simulink model "DDCU_wxt_v03"  (R2014a)
settings: Solver=ode45  StartTime=0.0  StopTime=50  FixedStep=0.0005  RelTol=1e-3
values from neighbouring files (symbols this model uses):
  ag_thr = 0.4*g    (= 3.924)    [Veh_Par_wxt.m]
  B = 2.25    [Veh_Par_wxt.m]
  bra_pre_em = 12    [Veh_Par_wxt.m]
  bra_pre_gz2 = 12/3    (= 4)    [Veh_Par_wxt.m]
  bra_pre_gz34 = 12/3    (= 4)    [Veh_Par_wxt.m]
  bra_pre_yd = 12/2    (= 6)    [Veh_Par_wxt.m]
  brakepre_dem_data = [0 1 2 3 4 5 6 7 8 9 10 11 12]    [Veh_Par_wxt.m]
  brakeTrq_dem_data = [0 218.198 436.396 654.594 872.792 1090.99 1309.188 1527.386 1745.584 1963.782 2181.98 2400.178 2618.376]    [Veh_Par_wxt.m]
  bratrq_max = 4*2618.376    (= 10473.504)    [Veh_Par_wxt.m]
  eff_tran = 0.75    [Veh_Par_wxt.m]
  G = Mass*g    (= 36297)    [Veh_Par_wxt.m]
  kd1 = 1    [Veh_Par_wxt.m]
  kd2 = 1    [Veh_Par_wxt.m]
  kd3 = 1    [Veh_Par_wxt.m]
  ki1 = 1    [Veh_Par_wxt.m]
  ki2 = 1    [Veh_Par_wxt.m]
  ki3 = 1    [Veh_Par_wxt.m]
  kp1 = 1    [Veh_Par_wxt.m]
  kp2 = 1    [Veh_Par_wxt.m]
  kp3 = 1    [Veh_Par_wxt.m]
  L = 3.12    [Veh_Par_wxt.m]
  premax = 12    [Veh_Par_wxt.m]
  Radius = 0.20    (= 0.2)    [Veh_Par_wxt.m]
  s_opt_yi_add = 0.05    [Veh_Par_wxt.m]
  s_opt_zhuan_add = 0.05    [Veh_Par_wxt.m]
  spd_map_mot = [0 100 200 300 360 400 500 600 700 800 900]*tras_ratio    [Veh_Par_wxt.m]
  spdmax = 900*tras_ratio    (= 5580)    [Veh_Par_wxt.m]
  speed_thr_park = 5/3.6/Radius*30/pi    (= 66.3145596216)    [Veh_Par_wxt.m]
  tras_ratio = 6.2    [Veh_Par_wxt.m]
  trq_map_mot = [1200 1200 1200 1200 1200 1080 864 720 617 540 480]/tras_ratio    [Veh_Par_wxt.m]
  trqmax = 80    [Veh_Par_wxt.m]
  v_thr1_b = 5    [Veh_Par_wxt.m]
  v_thr2_b = 20    [Veh_Par_wxt.m]
  v_thr_park = 5    [Veh_Par_wxt.m]
undefined symbols (not defined in the file or in its folder): DiscIntNeverNeededParam
libraries: simulink x34, Solver_SF x1
(part 7 of 10)

== system DDCU_wxt_v03/MainControl/mode_control/backward/backward/Drive/驱动防滑控制TCS/直行TCS/直行/Subsystem1 ==
  brake_dem : Inport
  1-D Lookup Table : Lookup_n-D  NumberOfTableDimensions=1  BreakpointsForDimension1=brakeTrq_dem_data  Table=brakepre_dem_data  InternalRulePriority=Speed  RndMeth=Simplest  InputSameDT=on
  Constant : Constant  Value=bratrq_max
  Gain1 : Gain  Gain=1/2
  Gain2 : Gain  Gain=1/100
  Gain3 : Gain  Gain=1/2
  Product : Product
  brakepre_dem : Outport
  wires:
  brake_dem/1 -> Gain2/1
  Gain3/1 -> 1-D Lookup Table/1
  Gain2/1 -> Product/2
  Gain1/1 -> Gain3/1
  Product/1 -> Gain1/1
  Constant/1 -> Product/1
  1-D Lookup Table/1 -> brakepre_dem/1

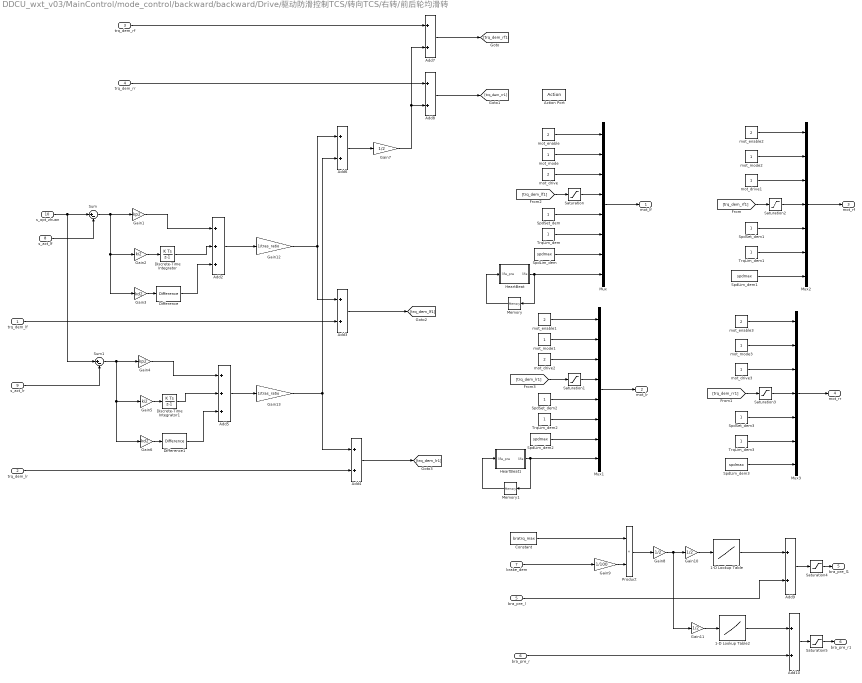
== system DDCU_wxt_v03/MainControl/mode_control/backward/backward/Drive/驱动防滑控制TCS/转向TCS/右转/前后轮均滑转 ==
  trq_dem_lf : Inport
  trq_dem_lr : Inport  Port=2
  trq_dem_rf : Inport  Port=3
  trq_dem_rr : Inport  Port=4
  bra_pre_l : Inport  Port=5
  bra_pre_r : Inport  Port=6
  brake_dem : Inport  Port=7
  s_act_lf : Inport  Port=8
  s_act_lr : Inport  Port=9
  s_opt_zhuan : Inport  Port=10
  Action Port : ActionPort
  1-D Lookup Table : Lookup_n-D  NumberOfTableDimensions=1  BreakpointsForDimension1=brakeTrq_dem_data  Table=brakepre_dem_data  InternalRulePriority=Speed  RndMeth=Simplest  InputSameDT=on
  1-D Lookup Table2 : Lookup_n-D  NumberOfTableDimensions=1  BreakpointsForDimension1=brakeTrq_dem_data  Table=brakepre_dem_data  InternalRulePriority=Speed  RndMeth=Simplest  InputSameDT=on
  Add{3..4,6..10} (7 alike) : Sum
  Add2 : Sum  Inputs=+++
  Add5 : Sum  Inputs=+++
  Constant : Constant  Value=bratrq_max
  Difference : simulink/Discrete/Difference  ICPrevInput=0.0  InputProcessing=Inherited  OutMin=[]  OutMax=[]  OutDataType=fixdt(1, 16)  OutScaling=2^-10  DoSatur=off
  Difference1 : simulink/Discrete/Difference  ICPrevInput=0.0  InputProcessing=Inherited  OutMin=[]  OutMax=[]  OutDataType=fixdt(1, 16)  OutScaling=2^-10  DoSatur=off
  Discrete-Time Integrator : DiscreteIntegrator  SampleTime=-1  ICPrevOutput=DiscIntNeverNeededParam  ICPrevScaledInput=DiscIntNeverNeededParam
  Discrete-Time Integrator1 : DiscreteIntegrator  SampleTime=-1  ICPrevOutput=DiscIntNeverNeededParam  ICPrevScaledInput=DiscIntNeverNeededParam
  Gain1 : Gain  Gain=kp2
  Gain{7..8,10..11} (4 alike) : Gain  Gain=1/2
  Gain12 : Gain  Gain=1/tras_ratio
  Gain13 : Gain  Gain=1/tras_ratio
  Gain2 : Gain  Gain=ki2
  Gain3 : Gain  Gain=kd2
  Gain4 : Gain  Gain=kp2
  Gain5 : Gain  Gain=ki2
  Gain6 : Gain  Gain=kd2
  Gain9 : Gain  Gain=1/100
  HeartBeat : MATLAB Function  TreatAsAtomicUnit=on
  HeartBeat1 : MATLAB Function  TreatAsAtomicUnit=on
  Memory : Memory  InheritSampleTime=on
  Memory1 : Memory  InheritSampleTime=on
  Mux : Mux  Inputs=8
  Mux1 : Mux  Inputs=8
  Mux2 : Mux  Inputs=7
  Mux3 : Mux  Inputs=7
  Product : Product
  Saturation{,1..3} (4 alike) : Saturate  UpperLimit=trqmax  LowerLimit=-trqmax
  Saturation4 : Saturate  UpperLimit=premax  LowerLimit=0
  Saturation5 : Saturate  UpperLimit=premax  LowerLimit=0
  SpdLim_dem{,1..3} (4 alike) : Constant  Value=spdmax
  SpdSet_dem{,1..3} (4 alike) : Constant
  Sum : Sum  Inputs=|+-
  Sum1 : Sum  Inputs=|+-
  TrqLim_dem{,1..3} (4 alike) : Constant
  mot_drive : Constant  Value=2
  mot_drive1 : Constant
  mot_drive2 : Constant  Value=2
  mot_drive3 : Constant
  mot_enable{,1..3} (4 alike) : Constant  Value=2
  mot_mode{,1..3} (4 alike) : Constant
  mot_lf : Outport
  mot_lr : Outport  Port=2
  mot_rf : Outport  Port=3
  mot_rr : Outport  Port=4
  bra_pre_l1 : Outport  Port=5
  bra_pre_r1 : Outport  Port=6
  wires:
  Saturation5/1 -> bra_pre_r1/1
  Saturation4/1 -> bra_pre_l1/1
  Saturation3/1 -> Mux3/4
  Saturation2/1 -> Mux2/4
  Saturation1/1 -> Mux1/4
  Saturation/1 -> Mux/4
  Difference1/1 -> Add5/3
  Discrete-Time Integrator1/1 -> Add5/2
  Difference/1 -> Add2/3
  Discrete-Time Integrator/1 -> Add2/2
  Gain3/1 -> Difference/1
  brake_dem/1 -> Gain9/1
  Add10/1 -> Saturation5/1
  bra_pre_r/1 -> Add10/2
  1-D Lookup Table2/1 -> Add10/1
  Gain11/1 -> 1-D Lookup Table2/1
  Gain10/1 -> 1-D Lookup Table/1
  Gain9/1 -> Product/2
  Gain8/1 -> Gain10/1, Gain11/1
  Product/1 -> Gain8/1
  Constant/1 -> Product/1
  1-D Lookup Table/1 -> Add9/1
  Add9/1 -> Saturation4/1
  bra_pre_l/1 -> Add9/2
  SpdLim_dem3/1 -> Mux3/7
  TrqLim_dem3/1 -> Mux3/6
  Mux3/1 -> mot_rr/1
  SpdSet_dem3/1 -> Mux3/5
  mot_enable3/1 -> Mux3/1
  [trq_dem_rr1] -> Saturation3/1
  mot_mode3/1 -> Mux3/2
  mot_drive3/1 -> Mux3/3
  SpdLim_dem2/1 -> Mux1/7
  Memory1/1 -> HeartBeat1/1(life_pre)
  HeartBeat1/1(life) -> Memory1/1, Mux1/8
  TrqLim_dem2/1 -> Mux1/6
  Mux1/1 -> mot_lr/1
  SpdSet_dem2/1 -> Mux1/5
  mot_enable1/1 -> Mux1/1
  [trq_dem_lr1] -> Saturation1/1
  mot_mode1/1 -> Mux1/2
  mot_drive2/1 -> Mux1/3
  SpdLim_dem1/1 -> Mux2/7
  TrqLim_dem1/1 -> Mux2/6
  Mux2/1 -> mot_rf/1
  SpdSet_dem1/1 -> Mux2/5
  mot_enable2/1 -> Mux2/1
  [trq_dem_rf1] -> Saturation2/1
  mot_mode2/1 -> Mux2/2
  mot_drive1/1 -> Mux2/3
  SpdLim_dem/1 -> Mux/7
  Memory/1 -> HeartBeat/1(life_pre)
  HeartBeat/1(life) -> Memory/1, Mux/8
  TrqLim_dem/1 -> Mux/6
  Mux/1 -> mot_lf/1
  SpdSet_dem/1 -> Mux/5
  mot_enable/1 -> Mux/1
  [trq_dem_lf1] -> Saturation/1
  mot_mode/1 -> Mux/2
  mot_drive/1 -> Mux/3
  s_opt_zhuan/1 -> Sum1/1, Sum/1
  Sum/1 -> Gain2/1, Gain3/1, Gain1/1
  Gain1/1 -> Add2/1
  Gain2/1 -> Discrete-Time Integrator/1
  s_act_lf/1 -> Sum/2
  Add2/1 -> Gain12/1
  trq_dem_lf/1 -> Add3/2
  Add3/1 -> [trq_dem_lf1]
  Add4/1 -> [trq_dem_lr1]
  Sum1/1 -> Gain5/1, Gain6/1, Gain4/1
  Gain4/1 -> Add5/1
  Gain5/1 -> Discrete-Time Integrator1/1
  Gain6/1 -> Difference1/1
  s_act_lr/1 -> Sum1/2
  Add5/1 -> Gain13/1
  trq_dem_lr/1 -> Add4/2
  Add6/1 -> Gain7/1
  trq_dem_rf/1 -> Add7/1
  Gain7/1 -> Add8/2, Add7/2
  Add7/1 -> [trq_dem_rf1]
  trq_dem_rr/1 -> Add8/1
  Add8/1 -> [trq_dem_rr1]
  Gain12/1 -> Add3/1, Add6/1
  Gain13/1 -> Add4/1, Add6/2

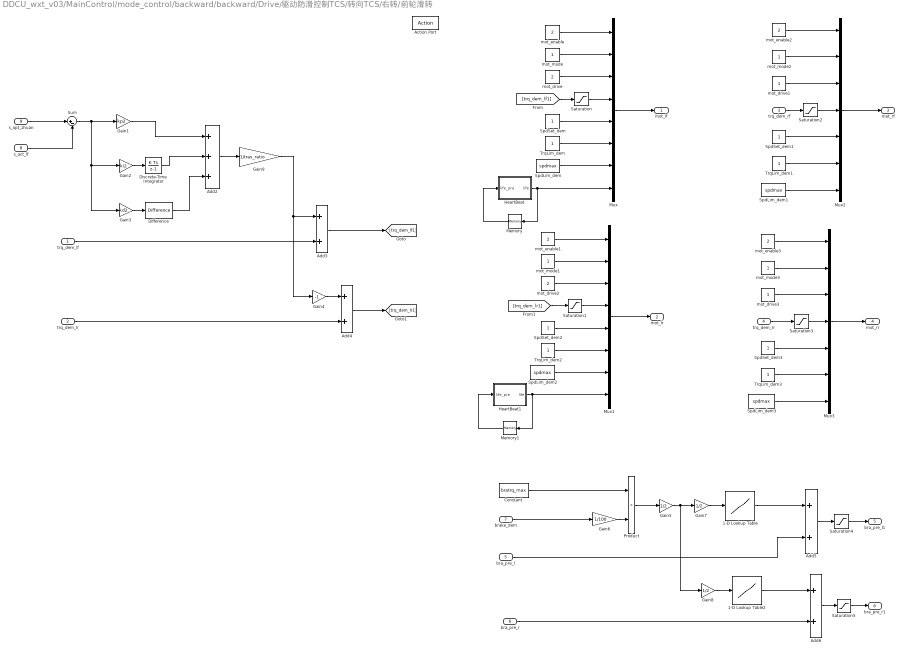
== system DDCU_wxt_v03/MainControl/mode_control/backward/backward/Drive/驱动防滑控制TCS/转向TCS/右转/前轮滑转 ==
  trq_dem_lf : Inport
  trq_dem_lr : Inport  Port=2
  trq_dem_rf : Inport  Port=3
  trq_dem_rr : Inport  Port=4
  bra_pre_l : Inport  Port=5
  bra_pre_r : Inport  Port=6
  brake_dem : Inport  Port=7
  s_act_lf : Inport  Port=8
  s_opt_zhuan : Inport  Port=9
  Action Port : ActionPort
  1-D Lookup Table : Lookup_n-D  NumberOfTableDimensions=1  BreakpointsForDimension1=brakeTrq_dem_data  Table=brakepre_dem_data  InternalRulePriority=Speed  RndMeth=Simplest  InputSameDT=on
  1-D Lookup Table2 : Lookup_n-D  NumberOfTableDimensions=1  BreakpointsForDimension1=brakeTrq_dem_data  Table=brakepre_dem_data  InternalRulePriority=Speed  RndMeth=Simplest  InputSameDT=on
  Add2 : Sum  Inputs=+++
  Add{3..6} (4 alike) : Sum
  Constant : Constant  Value=bratrq_max
  Difference : simulink/Discrete/Difference  ICPrevInput=0.0  InputProcessing=Inherited  OutMin=[]  OutMax=[]  OutDataType=fixdt(1, 16)  OutScaling=2^-10  DoSatur=off
  Discrete-Time Integrator : DiscreteIntegrator  SampleTime=-1  ICPrevOutput=DiscIntNeverNeededParam  ICPrevScaledInput=DiscIntNeverNeededParam
  Gain1 : Gain  Gain=kp2
  Gain2 : Gain  Gain=ki2
  Gain3 : Gain  Gain=kd2
  Gain4 : Gain  Gain=-1
  Gain5 : Gain  Gain=1/2
  Gain6 : Gain  Gain=1/100
  Gain7 : Gain  Gain=1/2
  Gain8 : Gain  Gain=1/2
  Gain9 : Gain  Gain=1/tras_ratio
  HeartBeat : MATLAB Function  TreatAsAtomicUnit=on
  HeartBeat1 : MATLAB Function  TreatAsAtomicUnit=on
  Memory : Memory  InheritSampleTime=on
  Memory1 : Memory  InheritSampleTime=on
  Mux : Mux  Inputs=8
  Mux1 : Mux  Inputs=8
  Mux2 : Mux  Inputs=7
  Mux3 : Mux  Inputs=7
  Product : Product
  Saturation{,1..3} (4 alike) : Saturate  UpperLimit=trqmax  LowerLimit=-trqmax
  Saturation4 : Saturate  UpperLimit=premax  LowerLimit=0
  Saturation5 : Saturate  UpperLimit=premax  LowerLimit=0
  SpdLim_dem{,1..3} (4 alike) : Constant  Value=spdmax
  SpdSet_dem{,1..3} (4 alike) : Constant
  Sum : Sum  Inputs=|+-
  TrqLim_dem{,1..3} (4 alike) : Constant
  mot_drive : Constant  Value=2
  mot_drive1 : Constant
  mot_drive2 : Constant  Value=2
  mot_drive3 : Constant
  mot_enable{,1..3} (4 alike) : Constant  Value=2
  mot_mode{,1..3} (4 alike) : Constant
  mot_lf : Outport
  mot_lr : Outport  Port=2
  mot_rf : Outport  Port=3
  mot_rr : Outport  Port=4
  bra_pre_l1 : Outport  Port=5
  bra_pre_r1 : Outport  Port=6
  wires:
  Saturation5/1 -> bra_pre_r1/1
  Saturation4/1 -> bra_pre_l1/1
  Saturation3/1 -> Mux3/4
  Saturation2/1 -> Mux2/4
  Saturation1/1 -> Mux1/4
  Saturation/1 -> Mux/4
  Difference/1 -> Add2/3
  Discrete-Time Integrator/1 -> Add2/2
  brake_dem/1 -> Gain6/1
  Add6/1 -> Saturation5/1
  bra_pre_r/1 -> Add6/2
  1-D Lookup Table2/1 -> Add6/1
  Gain8/1 -> 1-D Lookup Table2/1
  Gain7/1 -> 1-D Lookup Table/1
  Gain6/1 -> Product/2
  Gain5/1 -> Gain7/1, Gain8/1
  Product/1 -> Gain5/1
  Constant/1 -> Product/1
  1-D Lookup Table/1 -> Add5/1
  Add5/1 -> Saturation4/1
  bra_pre_l/1 -> Add5/2
  SpdLim_dem3/1 -> Mux3/7
  TrqLim_dem3/1 -> Mux3/6
  Mux3/1 -> mot_rr/1
  SpdSet_dem3/1 -> Mux3/5
  mot_enable3/1 -> Mux3/1
  trq_dem_rr/1 -> Saturation3/1
  mot_mode3/1 -> Mux3/2
  mot_drive3/1 -> Mux3/3
  SpdLim_dem2/1 -> Mux1/7
  Memory1/1 -> HeartBeat1/1(life_pre)
  HeartBeat1/1(life) -> Memory1/1, Mux1/8
  TrqLim_dem2/1 -> Mux1/6
  Mux1/1 -> mot_lr/1
  SpdSet_dem2/1 -> Mux1/5
  mot_enable1/1 -> Mux1/1
  [trq_dem_lr1] -> Saturation1/1
  mot_mode1/1 -> Mux1/2
  mot_drive2/1 -> Mux1/3
  SpdLim_dem1/1 -> Mux2/7
  TrqLim_dem1/1 -> Mux2/6
  Mux2/1 -> mot_rf/1
  SpdSet_dem1/1 -> Mux2/5
  mot_enable2/1 -> Mux2/1
  trq_dem_rf/1 -> Saturation2/1
  mot_mode2/1 -> Mux2/2
  mot_drive1/1 -> Mux2/3
  SpdLim_dem/1 -> Mux/7
  Memory/1 -> HeartBeat/1(life_pre)
  HeartBeat/1(life) -> Memory/1, Mux/8
  TrqLim_dem/1 -> Mux/6
  Mux/1 -> mot_lf/1
  SpdSet_dem/1 -> Mux/5
  mot_enable/1 -> Mux/1
  [trq_dem_lf1] -> Saturation/1
  mot_mode/1 -> Mux/2
  mot_drive/1 -> Mux/3
  s_opt_zhuan/1 -> Sum/1
  Sum/1 -> Gain2/1, Gain3/1, Gain1/1
  Gain1/1 -> Add2/1
  Gain2/1 -> Discrete-Time Integrator/1
  Gain3/1 -> Difference/1
  s_act_lf/1 -> Sum/2
  Add2/1 -> Gain9/1
  trq_dem_lf/1 -> Add3/2
  Add3/1 -> [trq_dem_lf1]
  Gain4/1 -> Add4/1
  trq_dem_lr/1 -> Add4/2
  Add4/1 -> [trq_dem_lr1]
  Gain9/1 -> Gain4/1, Add3/1

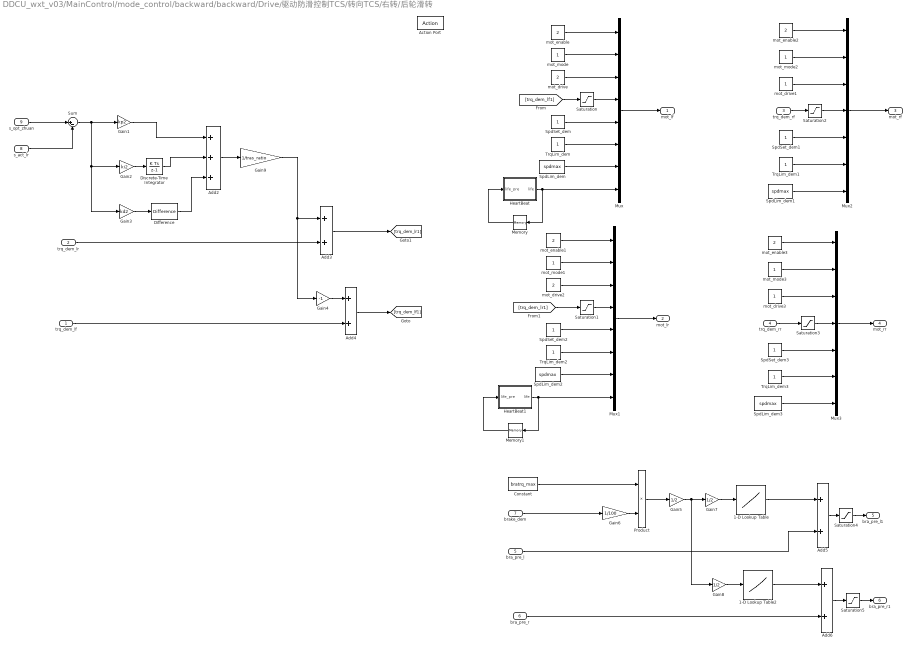
== system DDCU_wxt_v03/MainControl/mode_control/backward/backward/Drive/驱动防滑控制TCS/转向TCS/右转/后轮滑转 ==
  trq_dem_lf : Inport
  trq_dem_lr : Inport  Port=2
  trq_dem_rf : Inport  Port=3
  trq_dem_rr : Inport  Port=4
  bra_pre_l : Inport  Port=5
  bra_pre_r : Inport  Port=6
  brake_dem : Inport  Port=7
  s_act_lr : Inport  Port=8
  s_opt_zhuan : Inport  Port=9
  Action Port : ActionPort
  1-D Lookup Table : Lookup_n-D  NumberOfTableDimensions=1  BreakpointsForDimension1=brakeTrq_dem_data  Table=brakepre_dem_data  InternalRulePriority=Speed  RndMeth=Simplest  InputSameDT=on
  1-D Lookup Table2 : Lookup_n-D  NumberOfTableDimensions=1  BreakpointsForDimension1=brakeTrq_dem_data  Table=brakepre_dem_data  InternalRulePriority=Speed  RndMeth=Simplest  InputSameDT=on
  Add2 : Sum  Inputs=+++
  Add{3..6} (4 alike) : Sum
  Constant : Constant  Value=bratrq_max
  Difference : simulink/Discrete/Difference  ICPrevInput=0.0  InputProcessing=Inherited  OutMin=[]  OutMax=[]  OutDataType=fixdt(1, 16)  OutScaling=2^-10  DoSatur=off
  Discrete-Time Integrator : DiscreteIntegrator  SampleTime=-1  ICPrevOutput=DiscIntNeverNeededParam  ICPrevScaledInput=DiscIntNeverNeededParam
  Gain1 : Gain  Gain=kp2
  Gain2 : Gain  Gain=ki2
  Gain3 : Gain  Gain=kd2
  Gain4 : Gain  Gain=-1
  Gain5 : Gain  Gain=1/2
  Gain6 : Gain  Gain=1/100
  Gain7 : Gain  Gain=1/2
  Gain8 : Gain  Gain=1/2
  Gain9 : Gain  Gain=1/tras_ratio
  HeartBeat : MATLAB Function  TreatAsAtomicUnit=on
  HeartBeat1 : MATLAB Function  TreatAsAtomicUnit=on
  Memory : Memory  InheritSampleTime=on
  Memory1 : Memory  InheritSampleTime=on
  Mux : Mux  Inputs=8
  Mux1 : Mux  Inputs=8
  Mux2 : Mux  Inputs=7
  Mux3 : Mux  Inputs=7
  Product : Product
  Saturation{,1..3} (4 alike) : Saturate  UpperLimit=trqmax  LowerLimit=-trqmax
  Saturation4 : Saturate  UpperLimit=premax  LowerLimit=0
  Saturation5 : Saturate  UpperLimit=premax  LowerLimit=0
  SpdLim_dem{,1..3} (4 alike) : Constant  Value=spdmax
  SpdSet_dem{,1..3} (4 alike) : Constant
  Sum : Sum  Inputs=|+-
  TrqLim_dem{,1..3} (4 alike) : Constant
  mot_drive : Constant  Value=2
  mot_drive1 : Constant
  mot_drive2 : Constant  Value=2
  mot_drive3 : Constant
  mot_enable{,1..3} (4 alike) : Constant  Value=2
  mot_mode{,1..3} (4 alike) : Constant
  mot_lf : Outport
  mot_lr : Outport  Port=2
  mot_rf : Outport  Port=3
  mot_rr : Outport  Port=4
  bra_pre_l1 : Outport  Port=5
  bra_pre_r1 : Outport  Port=6
  wires:
  Saturation5/1 -> bra_pre_r1/1
  Saturation4/1 -> bra_pre_l1/1
  Saturation3/1 -> Mux3/4
  Saturation2/1 -> Mux2/4
  Saturation1/1 -> Mux1/4
  Saturation/1 -> Mux/4
  Difference/1 -> Add2/3
  Discrete-Time Integrator/1 -> Add2/2
  brake_dem/1 -> Gain6/1
  Add6/1 -> Saturation5/1
  bra_pre_r/1 -> Add6/2
  1-D Lookup Table2/1 -> Add6/1
  Gain8/1 -> 1-D Lookup Table2/1
  Gain7/1 -> 1-D Lookup Table/1
  Gain6/1 -> Product/2
  Gain5/1 -> Gain7/1, Gain8/1
  Product/1 -> Gain5/1
  Constant/1 -> Product/1
  1-D Lookup Table/1 -> Add5/1
  Add5/1 -> Saturation4/1
  bra_pre_l/1 -> Add5/2
  Add4/1 -> [trq_dem_lf1]
  trq_dem_lf/1 -> Add4/2
  Gain4/1 -> Add4/1
  Add3/1 -> [trq_dem_lr1]
  trq_dem_lr/1 -> Add3/2
  Add2/1 -> Gain9/1
  s_act_lr/1 -> Sum/2
  Gain3/1 -> Difference/1
  Gain2/1 -> Discrete-Time Integrator/1
  Gain1/1 -> Add2/1
  Sum/1 -> Gain1/1, Gain3/1, Gain2/1
  s_opt_zhuan/1 -> Sum/1
  mot_drive/1 -> Mux/3
  mot_mode/1 -> Mux/2
  [trq_dem_lf1] -> Saturation/1
  mot_enable/1 -> Mux/1
  SpdSet_dem/1 -> Mux/5
  Mux/1 -> mot_lf/1
  TrqLim_dem/1 -> Mux/6
  HeartBeat/1(life) -> Mux/8, Memory/1
  Memory/1 -> HeartBeat/1(life_pre)
  SpdLim_dem/1 -> Mux/7
  mot_drive1/1 -> Mux2/3
  mot_mode2/1 -> Mux2/2
  trq_dem_rf/1 -> Saturation2/1
  mot_enable2/1 -> Mux2/1
  SpdSet_dem1/1 -> Mux2/5
  Mux2/1 -> mot_rf/1
  TrqLim_dem1/1 -> Mux2/6
  SpdLim_dem1/1 -> Mux2/7
  mot_drive2/1 -> Mux1/3
  mot_mode1/1 -> Mux1/2
  [trq_dem_lr1] -> Saturation1/1
  mot_enable1/1 -> Mux1/1
  SpdSet_dem2/1 -> Mux1/5
  Mux1/1 -> mot_lr/1
  TrqLim_dem2/1 -> Mux1/6
  HeartBeat1/1(life) -> Mux1/8, Memory1/1
  Memory1/1 -> HeartBeat1/1(life_pre)
  SpdLim_dem2/1 -> Mux1/7
  mot_drive3/1 -> Mux3/3
  mot_mode3/1 -> Mux3/2
  trq_dem_rr/1 -> Saturation3/1
  mot_enable3/1 -> Mux3/1
  SpdSet_dem3/1 -> Mux3/5
  Mux3/1 -> mot_rr/1
  TrqLim_dem3/1 -> Mux3/6
  SpdLim_dem3/1 -> Mux3/7
  Gain9/1 -> Add3/1, Gain4/1

== system DDCU_wxt_v03/MainControl/mode_control/backward/backward/Drive/驱动防滑控制TCS/转向TCS/右转/无滑转 ==
  trq_dem_lf : Inport
  trq_dem_lr : Inport  Port=2
  trq_dem_rf : Inport  Port=3
  trq_dem_rr : Inport  Port=4
  bra_pre_l : Inport  Port=5
  bra_pre_r : Inport  Port=6
  brake_dem : Inport  Port=7
  Action Port : ActionPort
  1-D Lookup Table : Lookup_n-D  NumberOfTableDimensions=1  BreakpointsForDimension1=brakeTrq_dem_data  Table=brakepre_dem_data  InternalRulePriority=Speed  RndMeth=Simplest  InputSameDT=on
  1-D Lookup Table2 : Lookup_n-D  NumberOfTableDimensions=1  BreakpointsForDimension1=brakeTrq_dem_data  Table=brakepre_dem_data  InternalRulePriority=Speed  RndMeth=Simplest  InputSameDT=on
  Add2 : Sum
  Add3 : Sum
  Constant : Constant  Value=bratrq_max
  Gain1 : Gain  Gain=1/2
  Gain2 : Gain  Gain=1/100
  Gain3 : Gain  Gain=1/2
  Gain4 : Gain  Gain=1/2
  HeartBeat : MATLAB Function  TreatAsAtomicUnit=on
  HeartBeat1 : MATLAB Function  TreatAsAtomicUnit=on
  Memory : Memory  InheritSampleTime=on
  Memory1 : Memory  InheritSampleTime=on
  Mux : Mux  Inputs=8
  Mux1 : Mux  Inputs=8
  Mux2 : Mux  Inputs=7
  Mux3 : Mux  Inputs=7
  Product : Product
  Saturation{,1..3} (4 alike) : Saturate  UpperLimit=trqmax  LowerLimit=-trqmax
  Saturation4 : Saturate  UpperLimit=premax  LowerLimit=0
  Saturation5 : Saturate  UpperLimit=premax  LowerLimit=0
  SpdLim_dem{,1..3} (4 alike) : Constant  Value=spdmax
  SpdSet_dem{,1..3} (4 alike) : Constant
  TrqLim_dem{,1..3} (4 alike) : Constant
  mot_drive : Constant  Value=2
  mot_drive1 : Constant
  mot_drive2 : Constant  Value=2
  mot_drive3 : Constant
  mot_enable{,1..3} (4 alike) : Constant  Value=2
  mot_mode{,1..3} (4 alike) : Constant
  mot_lf : Outport
  mot_lr : Outport  Port=2
  mot_rf : Outport  Port=3
  mot_rr : Outport  Port=4
  bra_pre_l1 : Outport  Port=5
  bra_pre_r1 : Outport  Port=6
  wires:
  Saturation5/1 -> bra_pre_r1/1
  Saturation4/1 -> bra_pre_l1/1
  Saturation3/1 -> Mux3/4
  Saturation2/1 -> Mux2/4
  Saturation1/1 -> Mux1/4
  Saturation/1 -> Mux/4
  brake_dem/1 -> Gain2/1
  Add3/1 -> Saturation5/1
  bra_pre_r/1 -> Add3/2
  1-D Lookup Table2/1 -> Add3/1
  Gain4/1 -> 1-D Lookup Table2/1
  Gain3/1 -> 1-D Lookup Table/1
  Gain2/1 -> Product/2
  Gain1/1 -> Gain3/1, Gain4/1
  Product/1 -> Gain1/1
  Constant/1 -> Product/1
  1-D Lookup Table/1 -> Add2/1
  Add2/1 -> Saturation4/1
  bra_pre_l/1 -> Add2/2
  mot_drive/1 -> Mux/3
  mot_mode/1 -> Mux/2
  trq_dem_lf/1 -> Saturation/1
  mot_enable/1 -> Mux/1
  SpdSet_dem/1 -> Mux/5
  Mux/1 -> mot_lf/1
  TrqLim_dem/1 -> Mux/6
  HeartBeat/1(life) -> Mux/8, Memory/1
  Memory/1 -> HeartBeat/1(life_pre)
  SpdLim_dem/1 -> Mux/7
  mot_drive1/1 -> Mux2/3
  mot_mode2/1 -> Mux2/2
  trq_dem_rf/1 -> Saturation2/1
  mot_enable2/1 -> Mux2/1
  SpdSet_dem1/1 -> Mux2/5
  Mux2/1 -> mot_rf/1
  TrqLim_dem1/1 -> Mux2/6
  SpdLim_dem1/1 -> Mux2/7
  mot_drive2/1 -> Mux1/3
  mot_mode1/1 -> Mux1/2
  trq_dem_lr/1 -> Saturation1/1
  mot_enable1/1 -> Mux1/1
  SpdSet_dem2/1 -> Mux1/5
  Mux1/1 -> mot_lr/1
  TrqLim_dem2/1 -> Mux1/6
  HeartBeat1/1(life) -> Mux1/8, Memory1/1
  Memory1/1 -> HeartBeat1/1(life_pre)
  SpdLim_dem2/1 -> Mux1/7
  mot_drive3/1 -> Mux3/3
  mot_mode3/1 -> Mux3/2
  trq_dem_rr/1 -> Saturation3/1
  mot_enable3/1 -> Mux3/1
  SpdSet_dem3/1 -> Mux3/5
  Mux3/1 -> mot_rr/1
  TrqLim_dem3/1 -> Mux3/6
  SpdLim_dem3/1 -> Mux3/7

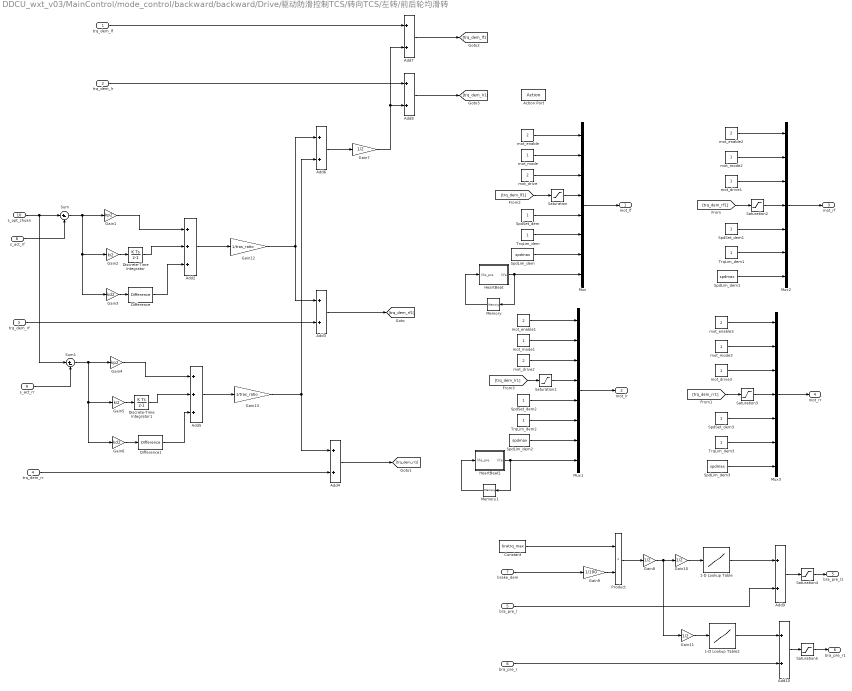
== system DDCU_wxt_v03/MainControl/mode_control/backward/backward/Drive/驱动防滑控制TCS/转向TCS/左转/前后轮均滑转 ==
  trq_dem_lf : Inport
  trq_dem_lr : Inport  Port=2
  trq_dem_rf : Inport  Port=3
  trq_dem_rr : Inport  Port=4
  bra_pre_l : Inport  Port=5
  bra_pre_r : Inport  Port=6
  brake_dem : Inport  Port=7
  s_act_rf : Inport  Port=8
  s_act_rr : Inport  Port=9
  s_opt_zhuan : Inport  Port=10
  Action Port : ActionPort
  1-D Lookup Table : Lookup_n-D  NumberOfTableDimensions=1  BreakpointsForDimension1=brakeTrq_dem_data  Table=brakepre_dem_data  InternalRulePriority=Speed  RndMeth=Simplest  InputSameDT=on
  1-D Lookup Table2 : Lookup_n-D  NumberOfTableDimensions=1  BreakpointsForDimension1=brakeTrq_dem_data  Table=brakepre_dem_data  InternalRulePriority=Speed  RndMeth=Simplest  InputSameDT=on
  Add{3..4,6..10} (7 alike) : Sum
  Add2 : Sum  Inputs=+++
  Add5 : Sum  Inputs=+++
  Constant : Constant  Value=bratrq_max
  Difference : simulink/Discrete/Difference  ICPrevInput=0.0  InputProcessing=Inherited  OutMin=[]  OutMax=[]  OutDataType=fixdt(1, 16)  OutScaling=2^-10  DoSatur=off
  Difference1 : simulink/Discrete/Difference  ICPrevInput=0.0  InputProcessing=Inherited  OutMin=[]  OutMax=[]  OutDataType=fixdt(1, 16)  OutScaling=2^-10  DoSatur=off
  Discrete-Time Integrator : DiscreteIntegrator  SampleTime=-1  ICPrevOutput=DiscIntNeverNeededParam  ICPrevScaledInput=DiscIntNeverNeededParam
  Discrete-Time Integrator1 : DiscreteIntegrator  SampleTime=-1  ICPrevOutput=DiscIntNeverNeededParam  ICPrevScaledInput=DiscIntNeverNeededParam
  Gain1 : Gain  Gain=kp2
  Gain{7..8,10..11} (4 alike) : Gain  Gain=1/2
  Gain12 : Gain  Gain=1/tras_ratio
  Gain13 : Gain  Gain=1/tras_ratio
  Gain2 : Gain  Gain=ki2
  Gain3 : Gain  Gain=kd2
  Gain4 : Gain  Gain=kp2
  Gain5 : Gain  Gain=ki2
  Gain6 : Gain  Gain=kd2
  Gain9 : Gain  Gain=1/100
  HeartBeat : MATLAB Function  TreatAsAtomicUnit=on
  HeartBeat1 : MATLAB Function  TreatAsAtomicUnit=on
  Memory : Memory  InheritSampleTime=on
  Memory1 : Memory  InheritSampleTime=on
  Mux : Mux  Inputs=8
  Mux1 : Mux  Inputs=8
  Mux2 : Mux  Inputs=7
  Mux3 : Mux  Inputs=7
  Product : Product
  Saturation{,1..3} (4 alike) : Saturate  UpperLimit=trqmax  LowerLimit=-trqmax
  Saturation4 : Saturate  UpperLimit=premax  LowerLimit=0
  Saturation5 : Saturate  UpperLimit=premax  LowerLimit=0
  SpdLim_dem{,1..3} (4 alike) : Constant  Value=spdmax
  SpdSet_dem{,1..3} (4 alike) : Constant
  Sum : Sum  Inputs=|+-
  Sum1 : Sum  Inputs=|+-
  TrqLim_dem{,1..3} (4 alike) : Constant
  mot_drive : Constant  Value=2
  mot_drive1 : Constant
  mot_drive2 : Constant  Value=2
  mot_drive3 : Constant
  mot_enable{,1..3} (4 alike) : Constant  Value=2
  mot_mode{,1..3} (4 alike) : Constant
  mot_lf : Outport
  mot_lr : Outport  Port=2
  mot_rf : Outport  Port=3
  mot_rr : Outport  Port=4
  bra_pre_l1 : Outport  Port=5
  bra_pre_r1 : Outport  Port=6
  wires:
  Saturation5/1 -> bra_pre_r1/1
  Saturation4/1 -> bra_pre_l1/1
  Saturation3/1 -> Mux3/4
  Saturation2/1 -> Mux2/4
  Saturation1/1 -> Mux1/4
  Saturation/1 -> Mux/4
  Difference1/1 -> Add5/3
  Discrete-Time Integrator1/1 -> Add5/2
  Difference/1 -> Add2/3
  Discrete-Time Integrator/1 -> Add2/2
  brake_dem/1 -> Gain9/1
  Add10/1 -> Saturation5/1
  bra_pre_r/1 -> Add10/2
  1-D Lookup Table2/1 -> Add10/1
  Gain11/1 -> 1-D Lookup Table2/1
  Gain10/1 -> 1-D Lookup Table/1
  Gain9/1 -> Product/2
  Gain8/1 -> Gain10/1, Gain11/1
  Product/1 -> Gain8/1
  Constant/1 -> Product/1
  1-D Lookup Table/1 -> Add9/1
  Add9/1 -> Saturation4/1
  bra_pre_l/1 -> Add9/2
  Add8/1 -> [trq_dem_lr1]
  trq_dem_lr/1 -> Add8/1
  Add7/1 -> [trq_dem_lf1]
  Gain7/1 -> Add7/2, Add8/2
  trq_dem_lf/1 -> Add7/1
  Add6/1 -> Gain7/1
  trq_dem_rr/1 -> Add4/2
  Add5/1 -> Gain13/1
  s_act_rr/1 -> Sum1/2
  Gain6/1 -> Difference1/1
  Gain5/1 -> Discrete-Time Integrator1/1
  Gain4/1 -> Add5/1
  Sum1/1 -> Gain4/1, Gain6/1, Gain5/1
  Add4/1 -> [trq_dem_rr1]
  Add3/1 -> [trq_dem_rf1]
  trq_dem_rf/1 -> Add3/2
  Add2/1 -> Gain12/1
  s_act_rf/1 -> Sum/2
  Gain3/1 -> Difference/1
  Gain2/1 -> Discrete-Time Integrator/1
  Gain1/1 -> Add2/1
  Sum/1 -> Gain1/1, Gain3/1, Gain2/1
  s_opt_zhuan/1 -> Sum/1, Sum1/1
  mot_drive/1 -> Mux/3
  mot_mode/1 -> Mux/2
  [trq_dem_lf1] -> Saturation/1
  mot_enable/1 -> Mux/1
  SpdSet_dem/1 -> Mux/5
  Mux/1 -> mot_lf/1
  TrqLim_dem/1 -> Mux/6
  HeartBeat/1(life) -> Mux/8, Memory/1
  Memory/1 -> HeartBeat/1(life_pre)
  SpdLim_dem/1 -> Mux/7
  mot_drive1/1 -> Mux2/3
  mot_mode2/1 -> Mux2/2
  [trq_dem_rf1] -> Saturation2/1
  mot_enable2/1 -> Mux2/1
  SpdSet_dem1/1 -> Mux2/5
  Mux2/1 -> mot_rf/1
  TrqLim_dem1/1 -> Mux2/6
  SpdLim_dem1/1 -> Mux2/7
  mot_drive2/1 -> Mux1/3
  mot_mode1/1 -> Mux1/2
  [trq_dem_lr1] -> Saturation1/1
  mot_enable1/1 -> Mux1/1
  SpdSet_dem2/1 -> Mux1/5
  Mux1/1 -> mot_lr/1
  TrqLim_dem2/1 -> Mux1/6
  HeartBeat1/1(life) -> Mux1/8, Memory1/1
  Memory1/1 -> HeartBeat1/1(life_pre)
  SpdLim_dem2/1 -> Mux1/7
  mot_drive3/1 -> Mux3/3
  mot_mode3/1 -> Mux3/2
  [trq_dem_rr1] -> Saturation3/1
  mot_enable3/1 -> Mux3/1
  SpdSet_dem3/1 -> Mux3/5
  Mux3/1 -> mot_rr/1
  TrqLim_dem3/1 -> Mux3/6
  SpdLim_dem3/1 -> Mux3/7
  Gain12/1 -> Add6/1, Add3/1
  Gain13/1 -> Add6/2, Add4/1

== system DDCU_wxt_v03/MainControl/mode_control/backward/backward/Drive/驱动防滑控制TCS/转向TCS/左转/前轮滑转 ==
  trq_dem_lf : Inport
  trq_dem_lr : Inport  Port=2
  trq_dem_rf : Inport  Port=3
  trq_dem_rr : Inport  Port=4
  bra_pre_l : Inport  Port=5
  bra_pre_r : Inport  Port=6
  brake_dem : Inport  Port=7
  s_act_rf : Inport  Port=8
  s_opt_zhuan : Inport  Port=9
  Action Port : ActionPort
  1-D Lookup Table : Lookup_n-D  NumberOfTableDimensions=1  BreakpointsForDimension1=brakeTrq_dem_data  Table=brakepre_dem_data  InternalRulePriority=Speed  RndMeth=Simplest  InputSameDT=on
  1-D Lookup Table2 : Lookup_n-D  NumberOfTableDimensions=1  BreakpointsForDimension1=brakeTrq_dem_data  Table=brakepre_dem_data  InternalRulePriority=Speed  RndMeth=Simplest  InputSameDT=on
  Add2 : Sum  Inputs=+++
  Add{3..6} (4 alike) : Sum
  Constant : Constant  Value=bratrq_max
  Difference : simulink/Discrete/Difference  ICPrevInput=0.0  InputProcessing=Inherited  OutMin=[]  OutMax=[]  OutDataType=fixdt(1, 16)  OutScaling=2^-10  DoSatur=off
  Discrete-Time Integrator : DiscreteIntegrator  SampleTime=-1  ICPrevOutput=DiscIntNeverNeededParam  ICPrevScaledInput=DiscIntNeverNeededParam
  Gain1 : Gain  Gain=kp2
  Gain2 : Gain  Gain=ki2
  Gain3 : Gain  Gain=kd2
  Gain4 : Gain  Gain=-1
  Gain5 : Gain  Gain=1/2
  Gain6 : Gain  Gain=1/100
  Gain7 : Gain  Gain=1/2
  Gain8 : Gain  Gain=1/2
  Gain9 : Gain  Gain=1/tras_ratio
  HeartBeat : MATLAB Function  TreatAsAtomicUnit=on
  HeartBeat1 : MATLAB Function  TreatAsAtomicUnit=on
  Memory : Memory  InheritSampleTime=on
  Memory1 : Memory  InheritSampleTime=on
  Mux : Mux  Inputs=8
  Mux1 : Mux  Inputs=8
  Mux2 : Mux  Inputs=7
  Mux3 : Mux  Inputs=7
  Product : Product
  Saturation{,1..3} (4 alike) : Saturate  UpperLimit=trqmax  LowerLimit=-trqmax
  Saturation4 : Saturate  UpperLimit=premax  LowerLimit=0
  Saturation5 : Saturate  UpperLimit=premax  LowerLimit=0
  SpdLim_dem{,1..3} (4 alike) : Constant  Value=spdmax
  SpdSet_dem{,1..3} (4 alike) : Constant
  Sum : Sum  Inputs=|+-
  TrqLim_dem{,1..3} (4 alike) : Constant
  mot_drive : Constant  Value=2
  mot_drive1 : Constant
  mot_drive2 : Constant  Value=2
  mot_drive3 : Constant
  mot_enable{,1..3} (4 alike) : Constant  Value=2
  mot_mode{,1..3} (4 alike) : Constant
  mot_lf : Outport
  mot_lr : Outport  Port=2
  mot_rf : Outport  Port=3
  mot_rr : Outport  Port=4
  bra_pre_l1 : Outport  Port=5
  bra_pre_r1 : Outport  Port=6
  wires:
  Saturation5/1 -> bra_pre_r1/1
  Saturation4/1 -> bra_pre_l1/1
  Saturation3/1 -> Mux3/4
  Saturation2/1 -> Mux2/4
  Saturation1/1 -> Mux1/4
  Saturation/1 -> Mux/4
  Difference/1 -> Add2/3
  Discrete-Time Integrator/1 -> Add2/2
  brake_dem/1 -> Gain6/1
  Add6/1 -> Saturation5/1
  bra_pre_r/1 -> Add6/2
  1-D Lookup Table2/1 -> Add6/1
  Gain8/1 -> 1-D Lookup Table2/1
  Gain7/1 -> 1-D Lookup Table/1
  Gain6/1 -> Product/2
  Gain5/1 -> Gain7/1, Gain8/1
  Product/1 -> Gain5/1
  Constant/1 -> Product/1
  1-D Lookup Table/1 -> Add5/1
  Add5/1 -> Saturation4/1
  bra_pre_l/1 -> Add5/2
  Add4/1 -> [trq_dem_rr1]
  trq_dem_rr/1 -> Add4/2
  Gain4/1 -> Add4/1
  Add3/1 -> [trq_dem_rf1]
  trq_dem_rf/1 -> Add3/2
  Add2/1 -> Gain9/1
  s_act_rf/1 -> Sum/2
  Gain3/1 -> Difference/1
  Gain2/1 -> Discrete-Time Integrator/1
  Gain1/1 -> Add2/1
  Sum/1 -> Gain1/1, Gain3/1, Gain2/1
  s_opt_zhuan/1 -> Sum/1
  mot_drive/1 -> Mux/3
  mot_mode/1 -> Mux/2
  trq_dem_lf/1 -> Saturation/1
  mot_enable/1 -> Mux/1
  SpdSet_dem/1 -> Mux/5
  Mux/1 -> mot_lf/1
  TrqLim_dem/1 -> Mux/6
  HeartBeat/1(life) -> Mux/8, Memory/1
  Memory/1 -> HeartBeat/1(life_pre)
  SpdLim_dem/1 -> Mux/7
  mot_drive1/1 -> Mux2/3
  mot_mode2/1 -> Mux2/2
  [trq_dem_rf1] -> Saturation2/1
  mot_enable2/1 -> Mux2/1
  SpdSet_dem1/1 -> Mux2/5
  Mux2/1 -> mot_rf/1
  TrqLim_dem1/1 -> Mux2/6
  SpdLim_dem1/1 -> Mux2/7
  mot_drive2/1 -> Mux1/3
  mot_mode1/1 -> Mux1/2
  trq_dem_lr/1 -> Saturation1/1
  mot_enable1/1 -> Mux1/1
  SpdSet_dem2/1 -> Mux1/5
  Mux1/1 -> mot_lr/1
  TrqLim_dem2/1 -> Mux1/6
  HeartBeat1/1(life) -> Mux1/8, Memory1/1
  Memory1/1 -> HeartBeat1/1(life_pre)
  SpdLim_dem2/1 -> Mux1/7
  mot_drive3/1 -> Mux3/3
  mot_mode3/1 -> Mux3/2
  [trq_dem_rr1] -> Saturation3/1
  mot_enable3/1 -> Mux3/1
  SpdSet_dem3/1 -> Mux3/5
  Mux3/1 -> mot_rr/1
  TrqLim_dem3/1 -> Mux3/6
  SpdLim_dem3/1 -> Mux3/7
  Gain9/1 -> Add3/1, Gain4/1

== system DDCU_wxt_v03/MainControl/mode_control/backward/backward/Drive/驱动防滑控制TCS/转向TCS/左转/后轮滑转 ==
  trq_dem_lf : Inport
  trq_dem_lr : Inport  Port=2
  trq_dem_rf : Inport  Port=3
  trq_dem_rr : Inport  Port=4
  bra_pre_l : Inport  Port=5
  bra_pre_r : Inport  Port=6
  brake_dem : Inport  Port=7
  s_act_rr : Inport  Port=8
  s_opt_zhuan : Inport  Port=9
  Action Port : ActionPort
  1-D Lookup Table : Lookup_n-D  NumberOfTableDimensions=1  BreakpointsForDimension1=brakeTrq_dem_data  Table=brakepre_dem_data  InternalRulePriority=Speed  RndMeth=Simplest  InputSameDT=on
  1-D Lookup Table2 : Lookup_n-D  NumberOfTableDimensions=1  BreakpointsForDimension1=brakeTrq_dem_data  Table=brakepre_dem_data  InternalRulePriority=Speed  RndMeth=Simplest  InputSameDT=on
  Add2 : Sum  Inputs=+++
  Add{3..6} (4 alike) : Sum
  Constant : Constant  Value=bratrq_max
  Difference : simulink/Discrete/Difference  ICPrevInput=0.0  InputProcessing=Inherited  OutMin=[]  OutMax=[]  OutDataType=fixdt(1, 16)  OutScaling=2^-10  DoSatur=off
  Discrete-Time Integrator : DiscreteIntegrator  SampleTime=-1  ICPrevOutput=DiscIntNeverNeededParam  ICPrevScaledInput=DiscIntNeverNeededParam
  Gain1 : Gain  Gain=kp2
  Gain2 : Gain  Gain=ki2
  Gain3 : Gain  Gain=kd2
  Gain4 : Gain  Gain=-1
  Gain5 : Gain  Gain=1/2
  Gain6 : Gain  Gain=1/100
  Gain7 : Gain  Gain=1/2
  Gain8 : Gain  Gain=1/2
  Gain9 : Gain  Gain=1/tras_ratio
  HeartBeat : MATLAB Function  TreatAsAtomicUnit=on
  HeartBeat1 : MATLAB Function  TreatAsAtomicUnit=on
  Memory : Memory  InheritSampleTime=on
  Memory1 : Memory  InheritSampleTime=on
  Mux : Mux  Inputs=8
  Mux1 : Mux  Inputs=8
  Mux2 : Mux  Inputs=7
  Mux3 : Mux  Inputs=7
  Product : Product
  Saturation{,1..3} (4 alike) : Saturate  UpperLimit=trqmax  LowerLimit=-trqmax
  Saturation4 : Saturate  UpperLimit=premax  LowerLimit=0
  Saturation5 : Saturate  UpperLimit=premax  LowerLimit=0
  SpdLim_dem{,1..3} (4 alike) : Constant  Value=spdmax
  SpdSet_dem{,1..3} (4 alike) : Constant
  Sum : Sum  Inputs=|+-
  TrqLim_dem{,1..3} (4 alike) : Constant
  mot_drive : Constant  Value=2
  mot_drive1 : Constant
  mot_drive2 : Constant  Value=2
  mot_drive3 : Constant
  mot_enable{,1..3} (4 alike) : Constant  Value=2
  mot_mode{,1..3} (4 alike) : Constant
  mot_lf : Outport
  mot_lr : Outport  Port=2
  mot_rf : Outport  Port=3
  mot_rr : Outport  Port=4
  bra_pre_l1 : Outport  Port=5
  bra_pre_r1 : Outport  Port=6
  wires:
  Saturation5/1 -> bra_pre_r1/1
  Saturation4/1 -> bra_pre_l1/1
  Saturation3/1 -> Mux3/4
  Saturation2/1 -> Mux1/4
  Saturation1/1 -> Mux2/4
  Saturation/1 -> Mux/4
  Difference/1 -> Add2/3
  Discrete-Time Integrator/1 -> Add2/2
  brake_dem/1 -> Gain6/1
  Add6/1 -> Saturation5/1
  bra_pre_r/1 -> Add6/2
  1-D Lookup Table2/1 -> Add6/1
  Gain8/1 -> 1-D Lookup Table2/1
  Gain7/1 -> 1-D Lookup Table/1
  Gain6/1 -> Product/2
  Gain5/1 -> Gain7/1, Gain8/1
  Product/1 -> Gain5/1
  Constant/1 -> Product/1
  1-D Lookup Table/1 -> Add5/1
  Add5/1 -> Saturation4/1
  bra_pre_l/1 -> Add5/2
  SpdLim_dem3/1 -> Mux3/7
  TrqLim_dem3/1 -> Mux3/6
  Mux3/1 -> mot_rr/1
  SpdSet_dem3/1 -> Mux3/5
  mot_enable3/1 -> Mux3/1
  [trq_dem_rr1] -> Saturation3/1
  mot_mode3/1 -> Mux3/2
  mot_drive3/1 -> Mux3/3
  SpdLim_dem2/1 -> Mux1/7
  Memory1/1 -> HeartBeat1/1(life_pre)
  HeartBeat1/1(life) -> Memory1/1, Mux1/8
  TrqLim_dem2/1 -> Mux1/6
  Mux1/1 -> mot_lr/1
  SpdSet_dem2/1 -> Mux1/5
  mot_enable1/1 -> Mux1/1
  trq_dem_lr/1 -> Saturation2/1
  mot_mode1/1 -> Mux1/2
  mot_drive2/1 -> Mux1/3
  SpdLim_dem1/1 -> Mux2/7
  TrqLim_dem1/1 -> Mux2/6
  Mux2/1 -> mot_rf/1
  SpdSet_dem1/1 -> Mux2/5
  mot_enable2/1 -> Mux2/1
  [trq_dem_rf1] -> Saturation1/1
  mot_mode2/1 -> Mux2/2
  mot_drive1/1 -> Mux2/3
  SpdLim_dem/1 -> Mux/7
  Memory/1 -> HeartBeat/1(life_pre)
  HeartBeat/1(life) -> Memory/1, Mux/8
  TrqLim_dem/1 -> Mux/6
  Mux/1 -> mot_lf/1
  SpdSet_dem/1 -> Mux/5
  mot_enable/1 -> Mux/1
  trq_dem_lf/1 -> Saturation/1
  mot_mode/1 -> Mux/2
  mot_drive/1 -> Mux/3
  s_opt_zhuan/1 -> Sum/1
  Sum/1 -> Gain2/1, Gain3/1, Gain1/1
  Gain1/1 -> Add2/1
  Gain2/1 -> Discrete-Time Integrator/1
  Gain3/1 -> Difference/1
  s_act_rr/1 -> Sum/2
  Add2/1 -> Gain9/1
  trq_dem_rr/1 -> Add3/2
  Add3/1 -> [trq_dem_rr1]
  Gain4/1 -> Add4/1
  trq_dem_rf/1 -> Add4/2
  Add4/1 -> [trq_dem_rf1]
  Gain9/1 -> Gain4/1, Add3/1

== system DDCU_wxt_v03/MainControl/mode_control/backward/backward/Drive/驱动防滑控制TCS/转向TCS/左转/无滑转 ==
  trq_dem_lf : Inport
  trq_dem_lr : Inport  Port=2
  trq_dem_rf : Inport  Port=3
  trq_dem_rr : Inport  Port=4
  bra_pre_l : Inport  Port=5
  bra_pre_r : Inport  Port=6
  brake_dem : Inport  Port=7
  Action Port : ActionPort
  1-D Lookup Table : Lookup_n-D  NumberOfTableDimensions=1  BreakpointsForDimension1=brakeTrq_dem_data  Table=brakepre_dem_data  InternalRulePriority=Speed  RndMeth=Simplest  InputSameDT=on
  1-D Lookup Table2 : Lookup_n-D  NumberOfTableDimensions=1  BreakpointsForDimension1=brakeTrq_dem_data  Table=brakepre_dem_data  InternalRulePriority=Speed  RndMeth=Simplest  InputSameDT=on
  Add : Sum
  Add2 : Sum
  Constant : Constant  Value=bratrq_max
  Gain1 : Gain  Gain=1/2
  Gain2 : Gain  Gain=1/100
  Gain3 : Gain  Gain=1/2
  Gain4 : Gain  Gain=1/2
  HeartBeat : MATLAB Function  TreatAsAtomicUnit=on
  HeartBeat1 : MATLAB Function  TreatAsAtomicUnit=on
  Memory : Memory  InheritSampleTime=on
  Memory1 : Memory  InheritSampleTime=on
  Mux : Mux  Inputs=8
  Mux1 : Mux  Inputs=8
  Mux2 : Mux  Inputs=7
  Mux3 : Mux  Inputs=7
  Product : Product
  Saturation{,1..3} (4 alike) : Saturate  UpperLimit=trqmax  LowerLimit=-trqmax
  Saturation4 : Saturate  UpperLimit=premax  LowerLimit=0
  Saturation5 : Saturate  UpperLimit=premax  LowerLimit=0
  SpdLim_dem{,1..3} (4 alike) : Constant  Value=spdmax
  SpdSet_dem{,1..3} (4 alike) : Constant
  TrqLim_dem{,1..3} (4 alike) : Constant
  mot_drive : Constant  Value=2
  mot_drive1 : Constant
  mot_drive2 : Constant  Value=2
  mot_drive3 : Constant
  mot_enable{,1..3} (4 alike) : Constant  Value=2
  mot_mode{,1..3} (4 alike) : Constant
  mot_lf : Outport
  mot_lr : Outport  Port=2
  mot_rf : Outport  Port=3
  mot_rr : Outport  Port=4
  bra_pre_l1 : Outport  Port=5
  bra_pre_r1 : Outport  Port=6
  wires:
  Saturation5/1 -> bra_pre_r1/1
  Saturation4/1 -> bra_pre_l1/1
  Saturation3/1 -> Mux3/4
  Saturation2/1 -> Mux2/4
  Saturation1/1 -> Mux1/4
  Saturation/1 -> Mux/4
  brake_dem/1 -> Gain2/1
  Add2/1 -> Saturation5/1
  bra_pre_r/1 -> Add2/2
  1-D Lookup Table2/1 -> Add2/1
  Gain4/1 -> 1-D Lookup Table2/1
  Gain3/1 -> 1-D Lookup Table/1
  Gain2/1 -> Product/2
  Gain1/1 -> Gain3/1, Gain4/1
  Product/1 -> Gain1/1
  Constant/1 -> Product/1
  1-D Lookup Table/1 -> Add/1
  Add/1 -> Saturation4/1
  bra_pre_l/1 -> Add/2
  SpdLim_dem3/1 -> Mux3/7
  TrqLim_dem3/1 -> Mux3/6
  Mux3/1 -> mot_rr/1
  SpdSet_dem3/1 -> Mux3/5
  mot_enable3/1 -> Mux3/1
  trq_dem_rr/1 -> Saturation3/1
  mot_mode3/1 -> Mux3/2
  mot_drive3/1 -> Mux3/3
  SpdLim_dem2/1 -> Mux1/7
  Memory1/1 -> HeartBeat1/1(life_pre)
  HeartBeat1/1(life) -> Memory1/1, Mux1/8
  TrqLim_dem2/1 -> Mux1/6
  Mux1/1 -> mot_lr/1
  SpdSet_dem2/1 -> Mux1/5
  mot_enable1/1 -> Mux1/1
  trq_dem_lr/1 -> Saturation1/1
  mot_mode1/1 -> Mux1/2
  mot_drive2/1 -> Mux1/3
  SpdLim_dem1/1 -> Mux2/7
  TrqLim_dem1/1 -> Mux2/6
  Mux2/1 -> mot_rf/1
  SpdSet_dem1/1 -> Mux2/5
  mot_enable2/1 -> Mux2/1
  trq_dem_rf/1 -> Saturation2/1
  mot_mode2/1 -> Mux2/2
  mot_drive1/1 -> Mux2/3
  SpdLim_dem/1 -> Mux/7
  Memory/1 -> HeartBeat/1(life_pre)
  HeartBeat/1(life) -> Memory/1, Mux/8
  TrqLim_dem/1 -> Mux/6
  Mux/1 -> mot_lf/1
  SpdSet_dem/1 -> Mux/5
  mot_enable/1 -> Mux/1
  trq_dem_lf/1 -> Saturation/1
  mot_mode/1 -> Mux/2
  mot_drive/1 -> Mux/3

== matlab function DDCU_wxt_v03/MainControl/mode_control/backward/backward/Drive/驱动防滑控制TCS/转向TCS/右转/MATLAB Function1 ==
  data: s_act_lr input; flag_lr output; s_opt_zhuan input; s_opt_zhuan_add input; flag_lr_pre input
function flag_lr = fcn(s_act_lr,s_opt_zhuan,s_opt_zhuan_add,flag_lr_pre)
%#codegen
if s_act_lr>s_opt_zhuan+s_opt_zhuan_add
    flag_lr=1;
elseif s_act_lr<s_opt_zhuan
    flag_lr = 0;
else
    flag_lr=flag_lr_pre;
end
end

== matlab function DDCU_wxt_v03/MainControl/mode_control/backward/backward/Drive/驱动防滑控制TCS/转向TCS/右转/前后轮均滑转/HeartBeat ==
  data: life_pre input; life output
function life = fcn(life_pre)
%#codegen
life=life_pre+1;
if life>15
    life=0;
end
end

== matlab function DDCU_wxt_v03/MainControl/mode_control/backward/backward/Drive/驱动防滑控制TCS/转向TCS/右转/前轮滑转/HeartBeat1 ==
  data: life_pre input; life output
function life = fcn(life_pre)
%#codegen
life=life_pre+1;
if life>15
    life=0;
end
end

== matlab function DDCU_wxt_v03/MainControl/mode_control/backward/backward/Drive/驱动防滑控制TCS/转向TCS/右转/无滑转/HeartBeat1 ==
  data: life_pre input; life output
function life = fcn(life_pre)
%#codegen
life=life_pre+1;
if life>15
    life=0;
end
end

== matlab function DDCU_wxt_v03/MainControl/mode_control/backward/backward/Drive/驱动防滑控制TCS/转向TCS/左转/MATLAB Function3 ==
  data: s_act_rr input; flag_rr output; s_opt_zhuan input; s_opt_zhuan_add input; flag_rr_pre input
function flag_rr = fcn(s_act_rr,s_opt_zhuan,s_opt_zhuan_add,flag_rr_pre)
%#codegen
if s_act_rr>s_opt_zhuan+s_opt_zhuan_add
    flag_rr=1;
elseif s_act_rr<s_opt_zhuan
    flag_rr = 0;
else
    flag_rr=flag_rr_pre;
end
end

== matlab function DDCU_wxt_v03/MainControl/mode_control/backward/backward/Drive/驱动防滑控制TCS/转向TCS/左转/前轮滑转/HeartBeat ==
  data: life_pre input; life output
function life = fcn(life_pre)
%#codegen
life=life_pre+1;
if life>15
    life=0;
end
end

== matlab function DDCU_wxt_v03/MainControl/mode_control/backward/backward/Drive/驱动防滑控制TCS/转向TCS/左转/无滑转/HeartBeat ==
  data: life_pre input; life output
function life = fcn(life_pre)
%#codegen
life=life_pre+1;
if life>15
    life=0;
end
end

== matlab function DDCU_wxt_v03/MainControl/mode_control/center_steer/center_steer/HeartBeat ==
  data: life_pre input; life output
function life = fcn(life_pre)
%#codegen
life=life_pre+1;
if life>15
    life=0;
end
end

== matlab function DDCU_wxt_v03/MainControl/mode_control/center_steer/center_steer/容错控制/MATLAB Function ==
  data: trq_dem_l input; trq_dem_lf output; trq_dem_r input; trqlim_lf input; trqlim_lr input; trqlim_rf input; trqlim_rr input; guzhang_lf input; guzhang_lr input; guzhang_rf input; guzhang_rr input; trq_dem_lr output; trq_dem_rf output; trq_dem_rr output; bra_pre_l output; bra_pre_r output; bra_pre_yd input; mode output
function [trq_dem_lf,trq_dem_lr,trq_dem_rf,trq_dem_rr,bra_pre_l,bra_pre_r,mode] = fcn(trq_dem_l,trq_dem_r,trqlim_lf,trqlim_lr,trqlim_rf,trqlim_rr,guzhang_lf,guzhang_lr,guzhang_rf,guzhang_rr,bra_pre_yd)
%#codegen
if guzhang_lf==0 && guzhang_lr==0 && guzhang_rf==0 && guzhang_rr==0    %0电机故障,平均分配
    trq_dem_lf=trq_dem_l/2;
    trq_dem_lr=trq_dem_l/2;
    trq_dem_rf=trq_dem_r/2;
    trq_dem_rr=trq_dem_r/2;
    bra_pre_l=0;
    bra_pre_r=0;
    mode=1;
elseif  guzhang_lf==1 && guzhang_lr==0 && guzhang_rf==0 && guzhang_rr==0  %1电机故障，同侧电机进行力矩转移,跟行车不同，对侧不降扭。
    trq_dem_lf=0;
    trq_dem_lr=min(trq_dem_l,trqlim_lr);
    trq_dem_rf=trq_dem_r/2;
    trq_dem_rr=trq_dem_r/2;
    bra_pre_l=0;
    bra_pre_r=0;
    mode=2;
elseif  guzhang_lf==0 && guzhang_lr==1 && guzhang_rf==0 && guzhang_rr==0
    trq_dem_lf=min(trq_dem_l,trqlim_lf);
    trq_dem_lr=0;
    trq_dem_rf=trq_dem_r/2;
    trq_dem_rr=trq_dem_r/2;
    bra_pre_l=0;
    bra_pre_r=0;
    mode=3;
elseif  guzhang_lf==0 && guzhang_lr==0 && guzhang_rf==1 && guzhang_rr==0
    trq_dem_rf=0;
    trq_dem_rr=min(trq_dem_r,trqlim_rr);
    trq_dem_lf=trq_dem_l/2;
    trq_dem_lr=trq_dem_l/2;
    bra_pre_l=0;
    bra_pre_r=0;
    mode=4;
elseif  guzhang_lf==0 && guzhang_lr==0 && guzhang_rf==0 && guzhang_rr==1
    trq_dem_rf=min(trq_dem_r,trqlim_rf);
    trq_dem_rr=0;
    trq_dem_lf=trq_dem_l/2;
    trq_dem_lr=trq_dem_l/2;
    bra_pre_l=0;
    bra_pre_r=0;
    mode=5;
elseif  guzhang_lf==1 && guzhang_lr==1 && guzhang_rf==0 && guzhang_rr==0  %2电机故障，左侧双电机故障，左侧履带施加制动，改为原地转向
    trq_dem_lf=0;
    trq_dem_lr=0;
    trq_dem_rf=trq_dem_r/2;
    trq_dem_rr=trq_dem_r/2;
    bra_pre_l=bra_pre_yd;
    bra_pre_r=0;
    mode=6;
elseif  guzhang_lf==0 && guzhang_lr==0 && guzhang_rf==1 && guzhang_rr==1  %右侧双电机故障
    trq_dem_lf=trq_dem_l/2;
    trq_dem_lr=trq_dem_l/2;
    trq_dem_rf=0;
    trq_dem_rr=0;
    bra_pre_l=0;
    bra_pre_r=bra_pre_yd;
    mode=7;
elseif  guzhang_lf==1 && guzhang_lr==0 && guzhang_rf==1 && guzhang_rr==0 %2电机故障，对侧双电机故障,有4种情况,前两电机故障
    trq_dem_lf=0;
    trq_dem_rf=0;
    trq_dem_lr=min(trq_dem_l,trqlim_lr);
    trq_dem_rr=min(trq_dem_r,trqlim_rr);
    bra_pre_l=0;
    bra_pre_r=0;
    mode=8;
elseif  guzhang_lf==0 && guzhang_lr==1 && guzhang_rf==0 && guzhang_rr==1 %后两电机故障
    trq_dem_lr=0;
    trq_dem_rr=0;
    trq_dem_lf=min(trq_dem_l,trqlim_lf);
    trq_dem_rf=min(trq_dem_r,trqlim_rf);
    bra_pre_l=0;
    bra_pre_r=0;
    mode=9;
elseif  guzhang_lf==1 && guzhang_lr==0 && guzhang_rf==0 && guzhang_rr==1 %左前电机和右后电机故障
    trq_dem_lf=0;
    trq_dem_rr=0;
    trq_dem_lr=min(trq_dem_l,trqlim_lr);
    trq_dem_rf=min(trq_dem_r,trqlim_rf);
    bra_pre_l=0;
    bra_pre_r=0;
    mode=10;
elseif  guzhang_lf==0 && guzhang_lr==1 && guzhang_rf==1 && guzhang_rr==0 %左后电机和右前电机故障
    trq_dem_lr=0;
    trq_dem_rf=0;
    trq_dem_lf=min(trq_dem_l,trqlim_lf);
    trq_dem_rr=min(trq_dem_r,trqlim_rr);
    bra_pre_l=0;
    bra_pre_r=0;
    mode=11;
elseif guzhang_lf==1 && guzhang_lr==1 && guzhang_rf==1 && guzhang_rr==0   % 三电机故障
    trq_dem_lf=0;
    trq_dem_lr=0;
    trq_dem_rf=0;
    trq_dem_rr=min(trq_dem_r,trqlim_rr);
    bra_pre_l=bra_pre_yd;
    bra_pre_r=0;
    mode=12;
elseif guzhang_lf==1 && guzhang_lr==1 && guzhang_rf==0 && guzhang_rr==1
    trq_dem_lf=0;
    trq_dem_lr=0;
    trq_dem_rf=min(trq_dem_r,trqlim_rf);
    trq_dem_rr=0;
    bra_pre_l=bra_pre_yd;
    bra_pre_r=0;
    mode=13;
elseif guzhang_lf==1 && guzhang_lr==0 && guzhang_rf==1 && guzhang_rr==1
    trq_dem_lf=0;
    trq_dem_lr=min(trq_dem_l,trqlim_lr);
    trq_dem_rf=0;
    trq_dem_rr=0;
    bra_pre_l=0;
    bra_pre_r=bra_pre_yd;
    mode=14;
elseif guzhang_lf==0 && guzhang_lr==1 && guzhang_rf==1 && guzhang_rr==1
    trq_dem_lf=min(trq_dem_l,trqlim_lf);
    trq_dem_lr=0;
    trq_dem_rf=0;
    trq_dem_rr=0;
    bra_pre_l=0;
    bra_pre_r=bra_pre_yd;
    mode=15;
else
    %     guzhang_lf==1 && guzhang_lr==1 && guzhang_rf==1 && guzhang_rr==1 %四电机故障
    trq_dem_lf=0;
    trq_dem_lr=0;
    trq_dem_rf=0;
    trq_dem_rr=0;
    bra_pre_l=0;
    bra_pre_r=0;
    mode=16;
end
trq_dem_lf=min(trqlim_lf,trq_dem_lf);trq_dem_lf=max(0,trq_dem_lf);
trq_dem_lr=min(trqlim_lr,trq_dem_lr);trq_dem_lr=max(0,trq_dem_lr);
trq_dem_rf=min(trqlim_rf,trq_dem_rf);trq_dem_rf=max(0,trq_dem_rf);
trq_dem_rr=min(trqlim_rr,trq_dem_rr);trq_dem_rr=max(0,trq_dem_rr);
bra_pre_l=bra_pre_l;
bra_pre_r=bra_pre_r;
end

== matlab function DDCU_wxt_v03/MainControl/mode_control/forward/forward/Drive/目标转向力矩确定模块/MATLAB Function ==
  data: steer_dem input; Rturn_min output; G input; L input; umax input; B input; Tpeak_L input; Tpeak_R input; eff_tran input; Radius input; f input
function Rturn_min = fcn(steer_dem,G,L,umax,B,Tpeak_L,Tpeak_R,eff_tran,Radius,f)
%#codegen
if steer_dem>0
    Rturn_min=(G*L*umax/(4*B*(Tpeak_R*eff_tran/Radius-f*G/2))-0.925)/0.15*B;
else
    Rturn_min=(G*L*umax/(4*B*(Tpeak_L*eff_tran/Radius-f*G/2))-0.925)/0.15*B;
end
end

== matlab function DDCU_wxt_v03/MainControl/mode_control/forward/forward/Drive/目标转向力矩确定模块/MATLAB Function1 ==
  data: v_act input; Rturn_min_ag output; ag_thr input
function Rturn_min_ag = fcn(v_act,ag_thr)
%#codegen

    Rturn_min_ag=(v_act/3.6)^2/ag_thr;
end

== matlab function DDCU_wxt_v03/MainControl/mode_control/forward/forward/Drive/目标转向力矩确定模块/MATLAB Function2 ==
  data: umax input; delta_Tsteer_max output; G input; L input; B input; Radius input; Rturn_min_xy input
function delta_Tsteer_max = fcn(umax,G,L,B,Radius,Rturn_min_xy)
%#codegen

    delta_Fsteer_max=umax/(0.925+0.15*(Rturn_min_xy/B))*G*L/(2*B);
    delta_Tsteer_max=delta_Fsteer_max*Radius;
    
end

== matlab function DDCU_wxt_v03/MainControl/mode_control/forward/forward/Drive/驱动防滑控制TCS/直行TCS/直行/HeartBeat1 ==
  data: life_pre input; life output
function life = fcn(life_pre)
%#codegen
life=life_pre+1;
if life>15
    life=0;
end
end

== matlab function DDCU_wxt_v03/MainControl/mode_control/forward/forward/Drive/驱动防滑控制TCS/直行TCS/直行/MATLAB Function1 ==
  data: s_act_lr input; flag_lr output; s_opt_zhuan input; s_opt_zhuan_add input; flag_lr_pre input
function flag_lr = fcn(s_act_lr,s_opt_zhuan,s_opt_zhuan_add,flag_lr_pre)
%#codegen
if s_act_lr>s_opt_zhuan+s_opt_zhuan_add
    flag_lr=1;
elseif s_act_lr<s_opt_zhuan
    flag_lr = 0;
else
    flag_lr=flag_lr_pre;
end
end

== matlab function DDCU_wxt_v03/MainControl/mode_control/forward/forward/Drive/驱动防滑控制TCS/直行TCS/直行/MATLAB Function3 ==
  data: s_act_rr input; flag_rr output; s_opt_zhuan input; s_opt_zhuan_add input; flag_rr_pre input
function flag_rr = fcn(s_act_rr,s_opt_zhuan,s_opt_zhuan_add,flag_rr_pre)
%#codegen
if s_act_rr>s_opt_zhuan+s_opt_zhuan_add
    flag_rr=1;
elseif s_act_rr<s_opt_zhuan
    flag_rr = 0;
else
    flag_rr=flag_rr_pre;
end
end

== matlab function DDCU_wxt_v03/MainControl/mode_control/forward/forward/Drive/驱动防滑控制TCS/转向TCS/MATLAB Function ==
  data: steer_dem input; y output
function y = fcn(steer_dem)
%#codegen左转为0，右转为1
if steer_dem>0
    y=0;
else
    y = 1;
end
end

== matlab function DDCU_wxt_v03/MainControl/mode_control/forward/forward/Drive/驱动防滑控制TCS/转向TCS/右转/MATLAB Function ==
  data: s_act_lf input; flag_lf output; s_opt_zhuan input; s_opt_zhuan_add input; flag_lf_pre input
function flag_lf = fcn(s_act_lf,s_opt_zhuan,s_opt_zhuan_add,flag_lf_pre)
%#codegen
if s_act_lf>s_opt_zhuan+s_opt_zhuan_add
    flag_lf=1;
elseif s_act_lf<s_opt_zhuan
    flag_lf = 0;
else
    flag_lf=flag_lf_pre;
end
end

== matlab function DDCU_wxt_v03/MainControl/mode_control/forward/forward/Drive/驱动防滑控制TCS/转向TCS/右转/MATLAB Function2 ==
  data: s_act_rf input; flag_rf output; s_opt_zhuan input; s_opt_zhuan_add input; flag_rf_pre input
function flag_rf = fcn(s_act_rf,s_opt_zhuan,s_opt_zhuan_add,flag_rf_pre)
%#codegen
if s_act_rf>s_opt_zhuan+s_opt_zhuan_add
    flag_rf=1;
elseif s_act_rf<s_opt_zhuan
    flag_rf = 0;
else
    flag_rf=flag_rf_pre;
end
end

== matlab function DDCU_wxt_v03/MainControl/mode_control/forward/forward/Drive/驱动防滑控制TCS/转向TCS/右转/MATLAB Function4 ==
  data: y output; flag_lf input; flag_lr input
function y = fcn(flag_lf,flag_lr)
%#codegen只判断外侧车轮滑转状况，不能满足要求再进一步修改。
if flag_lf==0 && flag_lr==0
    y=0;
elseif flag_lf==1 && flag_lr==0
    y=1;
elseif flag_lf==0 && flag_lr==1
    y=2;
else
    %     flag_lf==1 && flag_lr==1
    y=3;
end
end

== matlab function DDCU_wxt_v03/MainControl/mode_control/forward/forward/Drive/驱动防滑控制TCS/转向TCS/右转/前轮滑转/HeartBeat ==
  data: life_pre input; life output
function life = fcn(life_pre)
%#codegen
life=life_pre+1;
if life>15
    life=0;
end
end

== matlab function DDCU_wxt_v03/MainControl/mode_control/forward/forward/Drive/驱动防滑控制TCS/转向TCS/右转/后轮滑转/HeartBeat ==
  data: life_pre input; life output
function life = fcn(life_pre)
%#codegen
life=life_pre+1;
if life>15
    life=0;
end
end

== matlab function DDCU_wxt_v03/MainControl/mode_control/forward/forward/Drive/驱动防滑控制TCS/转向TCS/右转/无滑转/HeartBeat ==
  data: life_pre input; life output
function life = fcn(life_pre)
%#codegen
life=life_pre+1;
if life>15
    life=0;
end
end

== matlab function DDCU_wxt_v03/MainControl/mode_control/forward/forward/Drive/驱动防滑控制TCS/转向TCS/左转/MATLAB Function ==
  data: s_act_lf input; flag_lf output; s_opt_zhuan input; s_opt_zhuan_add input; flag_lf_pre input
function flag_lf = fcn(s_act_lf,s_opt_zhuan,s_opt_zhuan_add,flag_lf_pre)
%#codegen
if s_act_lf>s_opt_zhuan+s_opt_zhuan_add
    flag_lf=1;
elseif s_act_lf<s_opt_zhuan
    flag_lf = 0;
else
    flag_lf=flag_lf_pre;
end
end

== matlab function DDCU_wxt_v03/MainControl/mode_control/forward/forward/Drive/驱动防滑控制TCS/转向TCS/左转/MATLAB Function2 ==
  data: s_act_rf input; flag_rf output; s_opt_zhuan input; s_opt_zhuan_add input; flag_rf_pre input
function flag_rf = fcn(s_act_rf,s_opt_zhuan,s_opt_zhuan_add,flag_rf_pre)
%#codegen
if s_act_rf>s_opt_zhuan+s_opt_zhuan_add
    flag_rf=1;
elseif s_act_rf<s_opt_zhuan
    flag_rf = 0;
else
    flag_rf=flag_rf_pre;
end
end

== matlab function DDCU_wxt_v03/MainControl/mode_control/forward/forward/Drive/驱动防滑控制TCS/转向TCS/左转/MATLAB Function4 ==
  data: y output; flag_rf input; flag_rr input
function y = fcn(flag_rf,flag_rr)
%#codegen只判断外侧车轮滑转状况，不能满足要求再进一步修改。
if flag_rf==0 && flag_rr==0
    y=0;
elseif flag_rf==1 && flag_rr==0
    y=1;
elseif flag_rf==0 && flag_rr==1
    y=2;
else
    %     flag_rf==1 && flag_rr==1
    y=3;
end
end
